simulink model "ssc_battery_rom_qbat"  (R2021a)
settings: Solver=ode1be  StartTime=0.0  StopTime=3600  FixedStep=elec_dt  RelTol=1e-3
PreLoadFcn:
  | % Model parameters
  | ssc_battery_rom_qbat_param
undefined symbols (not defined in the file or in its folder): coolant_flow_qoff, coolant_flow_Toff, coolant_flow_Ton, elec_dt, heat_dt, iniBatteryTemp, iniCoolantTemp, R0_mat, sigbuilder_block, SOC_vec, T_vec, V0_mat
libraries: fl_lib x47, nesl_utility x47, ee_lib x14
(part 1 of 3)
CloseFcn:
  | clear iniBatterySOC iniBatteryTemp
  | clear T_vec AH_vec SOC_vec V0_mat R0_mat
  | clear R1_mat C1_mat Tau1_mat MdotCp
Description:
  | Battery With Heat Transfer Modeled with ROM from Q-Bat
settings Model: OrderedModelArguments=off  Creator=mkurzynka  LastModifiedBy=smiller
settings SolverCC: AlgebraicLoopSolver=TrustRegion
settings DataIOCC: ReturnWorkspaceOutputs=off  SignalLoggingName=logsout_ssc_battery_rom_qbat
settings DebuggingCC: SFMachineParentedDataDiag=warning  ArithmeticOperatorsInVariantConditions=warning
settings ModelReferenceCC: UpdateModelReferenceTargets=Force
settings SFSimCC: CustomCodeUndefinedFunction=UseInterfaceOnly
settings SimscapeCC: SimscapeLogType=all  SimscapeLogName=simlog_ssc_battery_rom_qbat

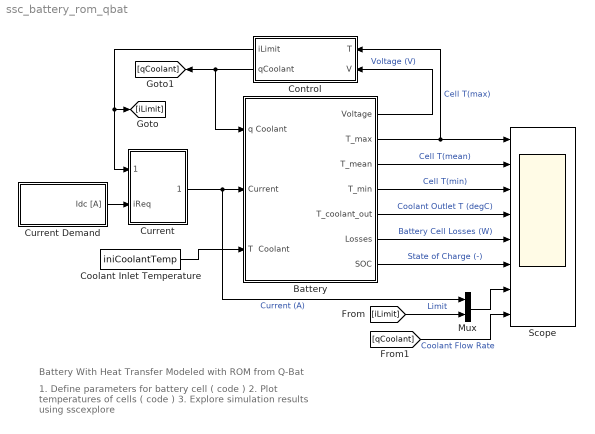
== system ssc_battery_rom_qbat ==
  note: Battery With Heat Transfer Modeled with ROM from Q-Bat
  note: 1. Define parameters for battery cell ( code )
      | 2. Plot temperatures of cells ( code )
      | 3. Explore simulation results using sscexplore
  Battery : Subsystem  mask(Electrothermal Battery Model){T_init_battery=iniBatteryTemp, T_init_th=iniCoolantTemp, Ts_thermal=heat_dt, Ts_electrical=elec_dt, n_maxsubiters=3, n_maxres=1e-3, solver_type=Iterative: PCG}
      mask prompts: T_init_battery "Battery Temperature (degC)"; T_init_th "Coolant Temperature (degC)"; Ts_thermal "Step size for thermal simulation"; Ts_electrical "Step size for electrical simulation"; n_maxsubiters "Number of thermal nonlinear subiterations"; n_maxres "Maximum error of thermal nonlinearity"; solver_type "Solver type"
      mask help:
      | Models a battery with temperature dependent behavior and heat transfer.
      |
      | The electrical behavior is modeled in Simscape, and consists of 14 cells connected in series.  Individual cells can be configured to have degraded behavior.
      |
      | The thermal behavior is a ROM exported from QBat.
      mask TypeOptions solver_type: Direct | Iterative: PCG
      mask DialogControl Container3 Prompt: Initial Conditions
      mask DialogControl Container4 Prompt: Simulation
      mask Display: image('ssc_battery_rom_qbat_battery.png');
  Control : Subsystem
  Coolant Inlet Temperature : Constant  Value=iniCoolantTemp
  Current : Subsystem
  Current Demand : Subsystem  Tag=STV Subsys  LoadFcn=sigbuilder_block('load');  StartFcn=sigbuilder_block('start');  StopFcn=sigbuilder_block('stop');  ClipboardFcn=sigbuilder_block('clipboard');  mask(Sigbuilder block){tuvar=[0:10]}
      mask help: Simulink:masks:SigbuilderBlock_MD
      mask init:
      | if ~strcmp(get_param(bdroot(gcbh),'SimulationStatus'),'stopped') tuvar = sigbuilder_block('maskInit'); end
      settings: CopyFcn=sigbuilder_block('copy');  DeleteFcn=sigbuilder_block('delete');  ModelCloseFcn=sigbuilder_block('modelClose');  PreSaveFcn=sigbuilder_block('preSave');  PauseFcn=sigbuilder_block('pause');  ContinueFcn=sigbuilder_block('continue');  NameChangeFcn=sigbuilder_block('namechange');  OpenFcn=sigbuilder_block('open',[207 275.4 463.8 230.4 ]);  CloseFcn=sigbuilder_block('close');
      mask Display: plot(0, 0, 100, 100,[2, 2, 32, 32, 2], [68, 8, 8, 68, 68],[32, 2], [38, 38], [32, 19, 2],[53, 60, 44], [32, 17, 17, 2],[16, 16, 31, 31]);txt = getActiveGroup(gcbh);text(2, 100, txt,'verticalAlignment', 'top');
  Mux : Mux  Inputs=2
  Scope : Scope  NumInputPorts=8
  wires:
  Battery/2(T_max) -> Scope/1, Control/1(T)  "Cell T(max)"
  Battery/3(T_mean) -> Scope/2  "Cell T(mean)"
  Battery/4(T_min) -> Scope/3  "Cell T(min)"
  Battery/7(SOC) -> Scope/6  "State of Charge (-)"
  Coolant Inlet Temperature/1 -> Battery/3(T  Coolant)
  Control/2(qCoolant) -> Battery/1(q Coolant), [qCoolant]
  Current/1(Current) -> Mux/1, Battery/2(Current)  "Current (A)"
  Battery/1(Voltage) -> Control/2(V)  "Voltage (V)"
  Battery/6(Losses) -> Scope/5  "Battery Cell Losses (W)"
  Current Demand/1(Idc [A]) -> Current/2(iReq)
  Mux/1 -> Scope/7
  [iLimit] -> Mux/2  "Limit"
  Control/1(iLimit) -> [iLimit], Current/1(iLimit)
  Battery/5(T_coolant_out) -> Scope/4  "Coolant Outlet T (degC)"
  [qCoolant] -> Scope/8  "Coolant Flow Rate"

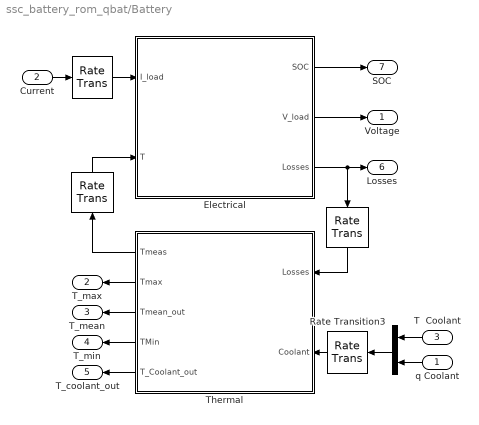
== system ssc_battery_rom_qbat/Battery ==
  q Coolant : Inport
  Current : Inport  Port=2
  T  Coolant : Inport  Port=3
  " " : RateTransition  OutPortSampleTime=elec_dt
  "  " : BusCreator  Inputs=2
  "   " : RateTransition  InitialCondition=0 * ones(14, 1)  OutPortSampleTime=Ts_thermal
  "    " : RateTransition  InitialCondition=(T_init_battery-273) * ones(14, 1)  OutPortSampleTime=Ts_electrical
  Electrical : Subsystem  mask(Electrical Behavior){init_battery_temp=T_init_battery, popup_faulted_cell=Cell 06, scale_factor_R0=1.2}
      mask prompts: init_battery_temp "Initial Battery Temperature (degK)"; popup_faulted_cell "Degraded Cell"; scale_factor_R0 "Scaling factor for terminal resistance for degraded cell"
      mask help: Models electrical behavior of battery. Select degraded cell and scale terminal resistance.
      mask init:
      | faulted_cell_str = get_param(gcb,'popup_faulted_cell');
      | for i = 1:14
      |     if i<10
      |         numstr = ['0' num2str(i)];
      |     else
      |         numstr = num2str(i);
      |     end
      | 
      |     set_param([gcb '/Cell ' numstr],'R0_mat','R0_mat');
      |     set_param([gcb '/Cell ' numstr],'BackgroundColor','[0.666667, 1.000000, 0.498039]');
      | end
      | if(~strcmpi(faulted_cell_str,'none'))
      |     set_param([gcb '/' faulted_cell_str],'R0_mat','R0_mat*scale_factor_R0');
      |     set_param([gcb '/' faulted_cell_str],'BackgroundColor','[1.000000, 0.600000, 0.600000]');
      | end
      mask TypeOptions popup_faulted_cell: None | Cell 01 | Cell 02 | Cell 03 | Cell 04 | Cell 05 | Cell 06 | Cell 07 | Cell 08 | Cell 09 | Cell 10 | Cell 11 | Cell 12 | Cell 13 | Cell 14
      mask Display: image('ssc_battery_rom_qbat_electrical.png');
  Rate Transition3 : RateTransition  InitialCondition=[iniCoolantTemp coolant_flow_qoff]  OutPortSampleTime=Ts_thermal
  Thermal : Subsystem
      mask Display: image('ssc_battery_rom_qbat_thermal.png');
  Voltage : Outport
  T_max : Outport  Port=2
  T_mean : Outport  Port=3
  T_min : Outport  Port=4
  T_coolant_out : Outport  Port=5
  Losses : Outport  Port=6
  SOC : Outport  Port=7
  wires:
  " "/1 -> Electrical/1(I_load)
  Electrical/3(Losses) -> "   "/1, Losses/1
  "  "/1 -> Rate Transition3/1
  Current/1 -> " "/1
  Electrical/1(SOC) -> SOC/1
  Electrical/2(V_load) -> Voltage/1
  T  Coolant/1 -> "  "/1
  q Coolant/1 -> "  "/2
  "    "/1 -> Electrical/2(T)
  "   "/1 -> Thermal/1(Losses)
  Rate Transition3/1 -> Thermal/2(Coolant)
  Thermal/1(Tmeas) -> "    "/1
  Thermal/2(Tmax) -> T_max/1
  Thermal/3(Tmean_out) -> T_mean/1
  Thermal/4(TMin) -> T_min/1
  Thermal/5(T_Coolant_out) -> T_coolant_out/1

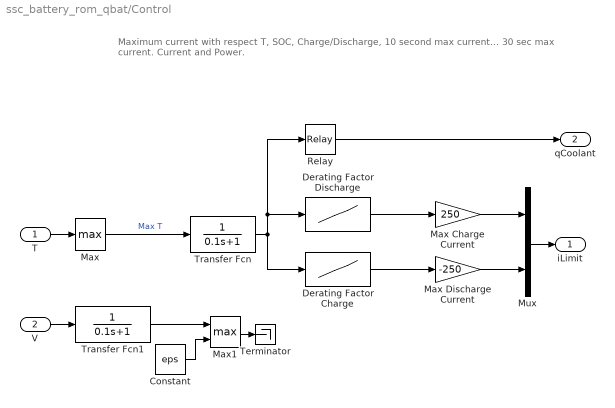
== system ssc_battery_rom_qbat/Control ==
  note: Maximum current with respect T, SOC, Charge/Discharge, 10 second max current... 30 sec max current. Current and Power.
  T : Inport
  V : Inport  Port=2
  Constant : Constant  Value=eps
  Derating Factor Charge : Lookup_n-D  NumberOfTableDimensions=1  BreakpointsForDimension1=[0 20 40 60]  Table=[1 1 1 0]  ExtrapMethod=Clip  UseLastTableValue=on  InternalRulePriority=Speed  RndMeth=Simplest  InputSameDT=on
  Derating Factor Discharge : Lookup_n-D  NumberOfTableDimensions=1  BreakpointsForDimension1=[0 20 40 60]  Table=[1 1 1 0]  ExtrapMethod=Clip  UseLastTableValue=on  InternalRulePriority=Speed  RndMeth=Simplest  InputSameDT=on
  Max : MinMax  Function=max
  Max Charge Current : Gain  Gain=250
  Max Discharge Current : Gain  Gain=-250
  Max1 : MinMax  Function=max  Inputs=2
  Mux : Mux  Inputs=2
  Relay : Relay  OnSwitchValue=coolant_flow_Ton  OffSwitchValue=coolant_flow_Toff  OnOutputValue=coolant_flow_qon  OffOutputValue=coolant_flow_qoff
  Terminator : Terminator
  Transfer Fcn : TransferFcn  Denominator=[0.1 1]
  Transfer Fcn1 : TransferFcn  Denominator=[0.1 1]
  iLimit : Outport
  qCoolant : Outport  Port=2
  wires:
  Transfer Fcn/1 -> Derating Factor Charge/1, Relay/1, Derating Factor Discharge/1
  Derating Factor Discharge/1 -> Max Charge Current/1
  Max Charge Current/1 -> Mux/1
  Transfer Fcn1/1 -> Max1/1
  Constant/1 -> Max1/2
  Relay/1 -> qCoolant/1
  T/1 -> Max/1
  V/1 -> Transfer Fcn1/1
  Max/1 -> Transfer Fcn/1  "Max T"
  Max1/1 -> Terminator/1
  Mux/1 -> iLimit/1
  Derating Factor Charge/1 -> Max Discharge Current/1
  Max Discharge Current/1 -> Mux/2

== system ssc_battery_rom_qbat/Current ==
  iLimit : Inport
  iReq : Inport  Port=2
  Demux : Demux  Outputs=2
  Min : MinMax  Inputs=2  ZeroCross=off
  Min1 : MinMax  Function=max  Inputs=2  ZeroCross=off
  Current : Outport
  wires:
  iReq/1 -> Min/2
  Demux/1 -> Min/1
  iLimit/1 -> Demux/1
  Min/1 -> Min1/1
  Demux/2 -> Min1/2
  Min1/1 -> Current/1

== system ssc_battery_rom_qbat/Current Demand ==
  Demux : Demux  Tag=STV Demux  Outputs=1
      settings: DisplayOption=none
  FromWs : FromWorkspace  Tag=STV FromWs  VariableName=tuvar
      SigBuilderData=|
      | common.afterFinalStr = 'Extrapolate'
      | common.sampleTime = 0
      | dataSet.timeRange = [0 3600]
      | dataSet.name = 'Drive Cycle 1'
      | sbobj.Groups.Name = 'Drive Cycle 1'
      | sbobj.Groups.Signals.Name = 'Idc [A]'
      | sbobj.Groups.Signals.XData = [0 0.421539907256 0.616158406753 0.810765207474 1.00512679999 1.19992814532 1.39456601073 1.58917271826 1.78373270062 1.97831601063 2.17292654009 2.36733272566 ... (18499 elements, 1x18499)]
      | sbobj.Groups.Signals.YData = [0 0 0 0 0 0 0 0 0 0 0 0 ... (18499 elements, 1x18499)]
      | sbobj.Groups.TimeRange = [0 3600]
  Idc [A] : Outport  Tag=STV Outport  VectorParamsAs1DForOutWhenUnconnected=off
  wires:
  FromWs/1 -> Demux/1
  Demux/1 -> Idc [A]/1
